simulink library "SUB_ECU_L4_MABX_HW_Interface_PTC_166"  (R2018a)
settings: Solver=VariableStepAuto  StartTime=0.0  StopTime=10.0  RelTol=1e-3
PostLoadFcn:
  | , if any(exist('dsrtsu_mdlpostloadfcn', 'file') == [2, 3, 6]), try dsrtsu_mdlpostloadfcn('Execute', bdroot); catch fprintf('Error in PostLoadFcn (dsrtsu_mdlpostloadfcn) for model "%s":\n %s\n', bdroot, lasterr); end, end,
undefined symbols (not defined in the file or in its folder): CANR_PROPB_REAX_3_13_CHANNEL_APV, CANR_PROPB_REAX_4_13_CHANNEL_APV, CANR_PROPB_XPR_1_50_CHANNEL_APV, ENUM_CAN_RX_T, ENUM_CAN_TX_T, ENUM_REAX_OPERATION_MODE_T, ENUM_SIGNAL_HEALTH_T, ENUM_XBR_CONTROL_MODE_T, ENUM_XBR_EBI_MODE_T, ENUM_XBR_PASS_THROUGH_ACTIVE_T, ENUM_XBR_PRIORITY_T, ENUM_XPR_INHIBIT_PARK_MANUAL_T, ENUM_XPR_INHIBIT_UNPARK_MANUAL_T, ENUM_XPR_PARK_MANUAL_T, ENUM_XPR_UNPARK_MANUAL_T, PROPB_REAX_1_E4_DES_POS_SIG_SRC_APV, PROPB_REAX_1_E4_DESIRED_OPMODE_APV, PROPB_REAX_1_E4_DESIRED_POSITION_APV, ptc_matlab_lib
libraries: PTC_MBDS_LIB x163, rtican x79, simulink x41, EmE_MBD_Blockset x35, rti1401lib_dio_type4 x8, simulink_need_slupdate x7, $bdroot x5, rti1401lib_adc_type4 x3, rtitasklib x1
(part 18 of 25)

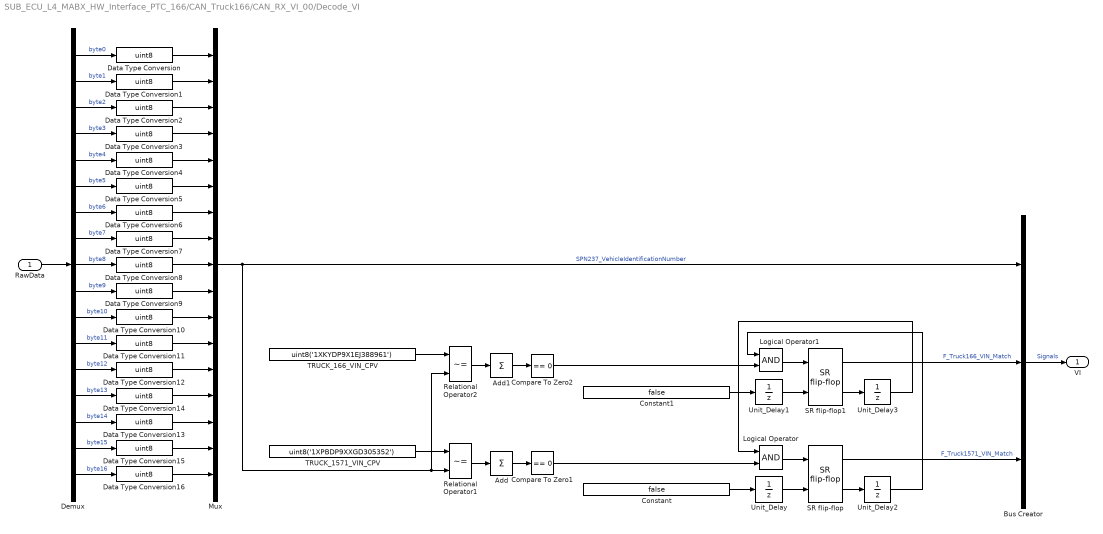
== system SUB_ECU_L4_MABX_HW_Interface_PTC_166/CAN_Truck166/CAN_RX_VI_00/Decode_VI ==
  RawData : Inport  OutDataTypeStr=uint8  PortDimensions=17
  Add : Sum  Inputs=+  InputSameDT=on
  Add1 : Sum  Inputs=+  InputSameDT=on
  Bus Creator : BusCreator  Inputs=3
  Compare To Zero1 : simulink/Logic and Bit Operations/Compare To Zero  relop===  OutDataTypeStr=boolean
  Compare To Zero2 : simulink/Logic and Bit Operations/Compare To Zero  relop===  OutDataTypeStr=boolean
  Constant : Constant  Value=false
  Constant1 : Constant  Value=false
  Data Type Conversion{,1..16} (17 alike) : DataTypeConversion  OutDataTypeStr=uint8
  Demux : Demux  Outputs=17
  Logical Operator : Logic  OutDataTypeStr=boolean
  Logical Operator1 : Logic  OutDataTypeStr=boolean
  Mux : Mux  Inputs=17
  Relational Operator1 : RelationalOperator  Operator=~=  OutDataTypeStr=boolean  RndMeth=Nearest  InputSameDT=on
  Relational Operator2 : RelationalOperator  Operator=~=  OutDataTypeStr=boolean  RndMeth=Nearest  InputSameDT=on
  SR flip-flop : EmE_MBD_Blockset/Logic and Bit Operations/SR flip-flop
      settings: SourceProductName=PACCAR EmE MBD Blockset
  SR flip-flop1 : EmE_MBD_Blockset/Logic and Bit Operations/SR flip-flop
      settings: SourceProductName=PACCAR EmE MBD Blockset
  TRUCK_1571_VIN_CPV : Constant  Value=uint8('1XPBDP9XXGD305352')
  TRUCK_166_VIN_CPV : Constant  Value=uint8('1XKYDP9X1EJ388961')
  Unit_Delay{,1..3} (4 alike) : UnitDelay  InitialCondition=true  SampleTime=-1
      settings: AttributesFormatString=IC: %<vinit>
  VI : Outport
  wires:
  Unit_Delay3/1 -> Logical Operator/1
  Unit_Delay2/1 -> Logical Operator1/1
  SR flip-flop/2 -> Unit_Delay2/1
  Compare To Zero2/1 -> Logical Operator1/2
  Logical Operator1/1 -> SR flip-flop1/1
  Logical Operator/1 -> SR flip-flop/1
  SR flip-flop1/2 -> Unit_Delay3/1
  Constant1/1 -> Unit_Delay1/1
  Unit_Delay1/1 -> SR flip-flop1/2
  Compare To Zero1/1 -> Logical Operator/2
  Constant/1 -> Unit_Delay/1
  Unit_Delay/1 -> SR flip-flop/2
  Bus Creator/1 -> VI/1  "Signals"
  Demux/17 -> Data Type Conversion16/1  "byte16"
  Demux/16 -> Data Type Conversion15/1  "byte15"
  Demux/1 -> Data Type Conversion/1  "byte0"
  Demux/15 -> Data Type Conversion13/1  "byte14"
  Demux/14 -> Data Type Conversion14/1  "byte13"
  Demux/2 -> Data Type Conversion1/1  "byte1"
  Demux/3 -> Data Type Conversion2/1  "byte2"
  Demux/13 -> Data Type Conversion12/1  "byte12"
  Demux/4 -> Data Type Conversion3/1  "byte3"
  Demux/12 -> Data Type Conversion11/1  "byte11"
  Demux/5 -> Data Type Conversion4/1  "byte4"
  Demux/11 -> Data Type Conversion10/1  "byte10"
  Demux/10 -> Data Type Conversion9/1  "byte9"
  Demux/6 -> Data Type Conversion5/1  "byte5"
  Demux/7 -> Data Type Conversion6/1  "byte6"
  Demux/9 -> Data Type Conversion8/1  "byte8"
  Demux/8 -> Data Type Conversion7/1  "byte7"
  SR flip-flop1/1 -> Bus Creator/2  "F_Truck166_VIN_Match"
  SR flip-flop/1 -> Bus Creator/3  "F_Truck1571_VIN_Match"
  Add1/1 -> Compare To Zero2/1
  Relational Operator2/1 -> Add1/1
  TRUCK_1571_VIN_CPV/1 -> Relational Operator1/1
  TRUCK_166_VIN_CPV/1 -> Relational Operator2/1
  Add/1 -> Compare To Zero1/1
  Relational Operator1/1 -> Add/1
  Data Type Conversion14/1 -> Mux/14
  Data Type Conversion4/1 -> Mux/5
  Data Type Conversion9/1 -> Mux/10
  Data Type Conversion3/1 -> Mux/4
  Data Type Conversion2/1 -> Mux/3
  Data Type Conversion15/1 -> Mux/16
  Data Type Conversion8/1 -> Mux/9
  Data Type Conversion13/1 -> Mux/15
  Data Type Conversion12/1 -> Mux/13
  Data Type Conversion7/1 -> Mux/8
  Data Type Conversion11/1 -> Mux/12
  Data Type Conversion10/1 -> Mux/11
  Data Type Conversion6/1 -> Mux/7
  Data Type Conversion1/1 -> Mux/2
  Data Type Conversion/1 -> Mux/1
  Data Type Conversion5/1 -> Mux/6
  Data Type Conversion16/1 -> Mux/17
  Mux/1 -> Bus Creator/1, Relational Operator1/2, Relational Operator2/2  "SPN237_VehicleIdentificationNumber"
  RawData/1 -> Demux/1

== system SUB_ECU_L4_MABX_HW_Interface_PTC_166/CAN_Truck166/Decode_PropB_REAX_3/decode_byte1 ==
  byte1 : Inport
  AND1 : PTC_MBDS_LIB/MBDS Standard Library/Basic Operations/Logic and Bit Operations/AND  BitwiseMode=on  Inputs=1  UseBitMask=on  BitMask=bin2dec('11110000')  OutDataTypeStr=uint8  PTC_MBDS_BlockVersion=5.41  PTC_BlockType=PTC_MBDS_AND
      settings: AttributesFormatString=bitwise  SourceProductName=PACCAR Technical Center MBDS Library
  AND2 : PTC_MBDS_LIB/MBDS Standard Library/Basic Operations/Logic and Bit Operations/AND  BitwiseMode=on  Inputs=1  UseBitMask=on  BitMask=bin2dec('00001111')  OutDataTypeStr=uint8  PTC_MBDS_BlockVersion=5.41  PTC_BlockType=PTC_MBDS_AND
      settings: AttributesFormatString=bitwise  SourceProductName=PACCAR Technical Center MBDS Library
  Bus Creator : BusCreator  Inputs=2
  "Shift_Arithmetic " : ArithShift  BitShiftNumber=4
  Out : Outport
  wires:
  Bus Creator/1 -> Out/1
  AND1/1 -> "Shift_Arithmetic "/1
  AND2/1 -> Bus Creator/1  "PropB_REAX_3_CurrentOperatingMode"
  byte1/1 -> AND2/1, AND1/1
  "Shift_Arithmetic "/1 -> Bus Creator/2  "PropB_REAX_3_ReqOperatingMode"

== system SUB_ECU_L4_MABX_HW_Interface_PTC_166/CAN_Truck166/Decode_PropB_REAX_3/decode_byte2 ==
  byte2 : Inport
  Bus Creator : BusCreator  Inputs=1
  Out : Outport
  wires:
  Bus Creator/1 -> Out/1
  byte2/1 -> Bus Creator/1  "PropB_REAX_3_StatusErrMsg"

== system SUB_ECU_L4_MABX_HW_Interface_PTC_166/CAN_Truck166/Decode_PropB_REAX_3/decode_byte3_byte4 ==
  byte3 : Inport
  byte4 : Inport  Port=2
  Bus Creator : BusCreator  Inputs=1
  Constant : Constant  Value=1/1024
  Data Type Conversion1 : DataTypeConversion  OutDataTypeStr=uint16  SaturateOnIntegerOverflow=on
  Data Type Conversion2 : DataTypeConversion  OutDataTypeStr=uint16  SaturateOnIntegerOverflow=on
  Data Type Conversion3 : DataTypeConversion  OutDataTypeStr=int16  ConvertRealWorld=Stored Integer (SI)
  Data Type Conversion4 : DataTypeConversion  SaturateOnIntegerOverflow=on
  OR : PTC_MBDS_LIB/MBDS Standard Library/Basic Operations/Logic and Bit Operations/OR  BitwiseMode=on  Inputs=2  UseBitMask=off  BitMask='A7'  OutDataTypeStr=uint16  PTC_MBDS_BlockVersion=5.41  PTC_BlockType=PTC_MBDS_OR
      settings: AttributesFormatString=bitwise  SourceProductName=PACCAR Technical Center MBDS Library
  Product : Product  Inputs=**  OutDataTypeStr=single  SaturateOnIntegerOverflow=on  InputSameDT=on
      settings: AttributesFormatString=Saturate: %<SaturateOnIntegerOverflow>
  Shift_Arithmetic 1 : ArithShift  BitShiftNumber=-8
  Out : Outport
  wires:
  Bus Creator/1 -> Out/1
  Data Type Conversion4/1 -> Product/1
  OR/1 -> Data Type Conversion3/1
  Shift_Arithmetic 1/1 -> OR/2
  Data Type Conversion1/1 -> OR/1
  Data Type Conversion2/1 -> Shift_Arithmetic 1/1
  byte4/1 -> Data Type Conversion2/1
  byte3/1 -> Data Type Conversion1/1
  Data Type Conversion3/1 -> Data Type Conversion4/1
  Constant/1 -> Product/2
  Product/1 -> Bus Creator/1  "PropB_REAX_3_HandwheelTorque"

== system SUB_ECU_L4_MABX_HW_Interface_PTC_166/CAN_Truck166/Decode_PropB_REAX_3/decode_byte5_byte6 ==
  byte5 : Inport
  byte6 : Inport  Port=2
  Bus Creator : BusCreator  Inputs=1
  Constant1 : Constant  Value=1/1024
  Data Type Conversion1 : DataTypeConversion  SaturateOnIntegerOverflow=on
  Data Type Conversion4 : DataTypeConversion  OutDataTypeStr=uint16  SaturateOnIntegerOverflow=on
  Data Type Conversion5 : DataTypeConversion  OutDataTypeStr=uint16  SaturateOnIntegerOverflow=on
  Data Type Conversion6 : DataTypeConversion  OutDataTypeStr=int16  ConvertRealWorld=Stored Integer (SI)
  OR1 : PTC_MBDS_LIB/MBDS Standard Library/Basic Operations/Logic and Bit Operations/OR  BitwiseMode=on  Inputs=2  UseBitMask=off  BitMask='A7'  OutDataTypeStr=uint16  PTC_MBDS_BlockVersion=5.41  PTC_BlockType=PTC_MBDS_OR
      settings: AttributesFormatString=bitwise  SourceProductName=PACCAR Technical Center MBDS Library
  Product1 : Product  Inputs=**  OutDataTypeStr=single  SaturateOnIntegerOverflow=on  InputSameDT=on
      settings: AttributesFormatString=Saturate: %<SaturateOnIntegerOverflow>
  Shift_Arithmetic 2 : ArithShift  BitShiftNumber=-8
  Out : Outport
  wires:
  Bus Creator/1 -> Out/1
  Data Type Conversion1/1 -> Product1/1
  Product1/1 -> Bus Creator/1  "PropB_REAX_3_HandwheelVelocity"
  Constant1/1 -> Product1/2
  Data Type Conversion6/1 -> Data Type Conversion1/1
  OR1/1 -> Data Type Conversion6/1
  Data Type Conversion4/1 -> OR1/1
  Data Type Conversion5/1 -> Shift_Arithmetic 2/1
  Shift_Arithmetic 2/1 -> OR1/2
  byte6/1 -> Data Type Conversion5/1
  byte5/1 -> Data Type Conversion4/1

== system SUB_ECU_L4_MABX_HW_Interface_PTC_166/CAN_Truck166/Decode_PropB_REAX_3/decode_byte7_byte8 ==
  byte7 : Inport
  byte8 : Inport  Port=2
  Bus Creator : BusCreator  Inputs=1
  Constant2 : Constant  Value=360/8192
  Data Type Conversion1 : DataTypeConversion  SaturateOnIntegerOverflow=on
  Data Type Conversion7 : DataTypeConversion  OutDataTypeStr=uint16  SaturateOnIntegerOverflow=on
  Data Type Conversion8 : DataTypeConversion  OutDataTypeStr=uint16  SaturateOnIntegerOverflow=on
  Data Type Conversion9 : DataTypeConversion  OutDataTypeStr=int16  ConvertRealWorld=Stored Integer (SI)
  OR2 : PTC_MBDS_LIB/MBDS Standard Library/Basic Operations/Logic and Bit Operations/OR  BitwiseMode=on  Inputs=2  UseBitMask=off  BitMask='A7'  OutDataTypeStr=uint16  PTC_MBDS_BlockVersion=5.41  PTC_BlockType=PTC_MBDS_OR
      settings: AttributesFormatString=bitwise  SourceProductName=PACCAR Technical Center MBDS Library
  Product2 : Product  Inputs=**  OutDataTypeStr=single  SaturateOnIntegerOverflow=on  InputSameDT=on
      settings: AttributesFormatString=Saturate: %<SaturateOnIntegerOverflow>
  Shift_Arithmetic 3 : ArithShift  BitShiftNumber=-8
  Out : Outport
  wires:
  Bus Creator/1 -> Out/1
  Data Type Conversion1/1 -> Product2/1
  Data Type Conversion9/1 -> Data Type Conversion1/1
  Constant2/1 -> Product2/2
  OR2/1 -> Data Type Conversion9/1
  Shift_Arithmetic 3/1 -> OR2/2
  Data Type Conversion7/1 -> OR2/1
  Data Type Conversion8/1 -> Shift_Arithmetic 3/1
  byte7/1 -> Data Type Conversion7/1
  Product2/1 -> Bus Creator/1  "PropB_REAX_3_PullCompensation"
  byte8/1 -> Data Type Conversion8/1

== system SUB_ECU_L4_MABX_HW_Interface_PTC_166/CAN_Truck166/Decode_PropB_REAX_4/decode_byte1 ==
  byte1 : Inport
  AND : PTC_MBDS_LIB/MBDS Standard Library/Basic Operations/Logic and Bit Operations/AND  BitwiseMode=on  Inputs=1  UseBitMask=on  BitMask=bin2dec('00000001')  OutDataTypeStr=boolean  PTC_MBDS_BlockVersion=5.41  PTC_BlockType=PTC_MBDS_AND
      settings: AttributesFormatString=bitwise  SourceProductName=PACCAR Technical Center MBDS Library
  AND1 : PTC_MBDS_LIB/MBDS Standard Library/Basic Operations/Logic and Bit Operations/AND  BitwiseMode=on  Inputs=1  UseBitMask=on  BitMask=bin2dec('00000010')  OutDataTypeStr=uint8  PTC_MBDS_BlockVersion=5.41  PTC_BlockType=PTC_MBDS_AND
      settings: AttributesFormatString=bitwise  SourceProductName=PACCAR Technical Center MBDS Library
  AND2 : PTC_MBDS_LIB/MBDS Standard Library/Basic Operations/Logic and Bit Operations/AND  BitwiseMode=on  Inputs=1  UseBitMask=on  BitMask=bin2dec('00000100')  OutDataTypeStr=uint8  PTC_MBDS_BlockVersion=5.41  PTC_BlockType=PTC_MBDS_AND
      settings: AttributesFormatString=bitwise  SourceProductName=PACCAR Technical Center MBDS Library
  Bus Creator : BusCreator  Inputs=3
  Data Type Conversion : DataTypeConversion  OutDataTypeStr=boolean  SaturateOnIntegerOverflow=on
  Data Type Conversion1 : DataTypeConversion  OutDataTypeStr=boolean  SaturateOnIntegerOverflow=on
  "Shift_Arithmetic " : ArithShift  BitShiftNumber=1
  Shift_Arithmetic 1 : ArithShift  BitShiftNumber=2
  Out : Outport
  wires:
  Data Type Conversion1/1 -> Bus Creator/3  "PropB_REAX_4_DriverControlledEffortsEnabled"
  Data Type Conversion/1 -> Bus Creator/2  "PropB_REAX_4_PositionIndexValid"
  Bus Creator/1 -> Out/1
  Shift_Arithmetic 1/1 -> Data Type Conversion1/1
  "Shift_Arithmetic "/1 -> Data Type Conversion/1
  AND1/1 -> "Shift_Arithmetic "/1
  byte1/1 -> AND/1, AND1/1, AND2/1
  AND2/1 -> Shift_Arithmetic 1/1
  AND/1 -> Bus Creator/1  "PropB_REAX_4_AbsSteeringPosValid"

== system SUB_ECU_L4_MABX_HW_Interface_PTC_166/CAN_Truck166/Decode_PropB_REAX_4/decode_byte2 ==
  byte2 : Inport
  Bus Creator : BusCreator  Inputs=1
  SignalConversion : SignalConversion  ConversionOutput=Contiguous copy  OverrideOpt=off
  Out : Outport
  wires:
  Bus Creator/1 -> Out/1
  SignalConversion/1 -> Bus Creator/1  "PropB_REAX_4_ControlOperatingMode"
  byte2/1 -> SignalConversion/1

== system SUB_ECU_L4_MABX_HW_Interface_PTC_166/CAN_Truck166/Decode_PropB_REAX_4/decode_byte3 ==
  byte3 : Inport
  Bus Creator : BusCreator  Inputs=1
  SignalConversion : SignalConversion  ConversionOutput=Contiguous copy  OverrideOpt=off
  Out : Outport
  wires:
  Bus Creator/1 -> Out/1
  SignalConversion/1 -> Bus Creator/1  "PropB_REAX_4_SystemMode"
  byte3/1 -> SignalConversion/1

== system SUB_ECU_L4_MABX_HW_Interface_PTC_166/CAN_Truck166/Decode_PropB_REAX_4/decode_byte5 ==
  byte5 : Inport
  Bus Creator : BusCreator  Inputs=1
  Data Type Conversion4 : DataTypeConversion  OutDataTypeStr=int8  ConvertRealWorld=Stored Integer (SI)
  Data Type Conversion5 : DataTypeConversion  OutDataTypeStr=double  SaturateOnIntegerOverflow=on
  Out : Outport
  wires:
  Bus Creator/1 -> Out/1
  Data Type Conversion5/1 -> Bus Creator/1  "PropB_REAX_4_PercHandwheelTorque"
  Data Type Conversion4/1 -> Data Type Conversion5/1
  byte5/1 -> Data Type Conversion4/1

== system SUB_ECU_L4_MABX_HW_Interface_PTC_166/CAN_Truck166/Decode_PropB_REAX_4/decode_byte6_byte7 ==
  byte6 : Inport
  byte7 : Inport  Port=2
  Bus Creator : BusCreator  Inputs=1
  Data Type Conversion6 : DataTypeConversion  OutDataTypeStr=uint16  SaturateOnIntegerOverflow=on
  Data Type Conversion7 : DataTypeConversion  OutDataTypeStr=uint16  SaturateOnIntegerOverflow=on
  Data Type Conversion8 : DataTypeConversion  OutDataTypeStr=int16  ConvertRealWorld=Stored Integer (SI)
  Data Type Conversion9 : DataTypeConversion  OutDataTypeStr=double  SaturateOnIntegerOverflow=on
  OR : PTC_MBDS_LIB/MBDS Standard Library/Basic Operations/Logic and Bit Operations/OR  BitwiseMode=on  Inputs=2  UseBitMask=off  BitMask='A7'  OutDataTypeStr=uint16  PTC_MBDS_BlockVersion=5.41  PTC_BlockType=PTC_MBDS_OR
      settings: AttributesFormatString=bitwise  SourceProductName=PACCAR Technical Center MBDS Library
  Shift_Arithmetic 2 : ArithShift  BitShiftNumber=-8
  Out : Outport
  wires:
  Bus Creator/1 -> Out/1
  OR/1 -> Data Type Conversion8/1
  Data Type Conversion8/1 -> Data Type Conversion9/1
  Shift_Arithmetic 2/1 -> OR/2
  Data Type Conversion7/1 -> Shift_Arithmetic 2/1
  Data Type Conversion6/1 -> OR/1
  byte7/1 -> Data Type Conversion7/1
  byte6/1 -> Data Type Conversion6/1
  Data Type Conversion9/1 -> Bus Creator/1  "PropB_REAX_4_AbsSteeringAngle"

== system SUB_ECU_L4_MABX_HW_Interface_PTC_166/CAN_Truck166/Decode_PropB_REAX_4/decode_byte8 ==
  byte8 : Inport
  Bus Creator : BusCreator  Inputs=1
  Data Type Conversion10 : DataTypeConversion  OutDataTypeStr=int8  ConvertRealWorld=Stored Integer (SI)
  Data Type Conversion11 : DataTypeConversion  OutDataTypeStr=double  SaturateOnIntegerOverflow=on
  Out : Outport
  wires:
  Bus Creator/1 -> Out/1
  byte8/1 -> Data Type Conversion10/1
  Data Type Conversion10/1 -> Data Type Conversion11/1
  Data Type Conversion11/1 -> Bus Creator/1  "PropB_REAX_4_PercMotorTorque"

== system SUB_ECU_L4_MABX_HW_Interface_PTC_166/DIGITAL/PWM pedal input management/Arbitrate pedal position output ==
  F_Pedal_pwm_sens_total_failure : Inport
  Pedal_synch_data_F_Hard : Inport  Port=2
  Pedal_pwm_angle_common : Inport  Port=3
  CPV : EmE_MBD_Blockset/Sources/CPV  conval=0.1
      settings: SourceProductName=PACCAR EmE MBD Blockset
  F_PEDAL_TORQUE_SLEW_AT_FAULT : Constant  Value=true
  If_Then_Else : EmE_MBD_Blockset/Signal Routing/If_Then_Else
      settings: SourceProductName=PACCAR EmE MBD Blockset
  Logical Operator1 : Logic  Operator=OR  OutDataTypeStr=boolean
  Logical Operator6 : Logic  Operator=OR  OutDataTypeStr=boolean
  PEDAL_PWM_SENSOR_DATA_APV.DEFAULT_SLEW_DOWN : Constant  Value=25
  PEDAL_PWM_SENSOR_DATA_APV.DEFAULT_SLEW_UP : Constant  Value=25
  PEDAL_PWM_SENSOR_DATA_APV.DEFAULT_VALUE : Constant  Value=0
  PEDAL_PWM_SENSOR_DATA_APV.DT : Constant  Value=0.01
  Relational Operator : EmE_MBD_Blockset/Logic and Bit Operations/Relational Operator  func=<=
      settings: SourceProductName=PACCAR EmE MBD Blockset
  SR flip-flop1 : EmE_MBD_Blockset/Logic and Bit Operations/SR flip-flop
      settings: SourceProductName=PACCAR EmE MBD Blockset
  Slew_at_event : EmE_MBD_Blockset/Math Operators/Slew_at_event
      settings: SourceProductName=PACCAR EmE MBD Blockset
  Terminator : Terminator
  Pedal_pwm_position : Outport
  DEFAULT_VALUE : Outport  Port=2
  wires:
  F_Pedal_pwm_sens_total_failure/1 -> Logical Operator6/1
  Slew_at_event/1 -> Logical Operator1/2
  CPV/1 -> Relational Operator/2
  SR flip-flop1/1 -> If_Then_Else/1
  SR flip-flop1/2 -> Terminator/1
  Logical Operator1/1 -> SR flip-flop1/1  "F_Pedal_pwm_fault_slew_enabled"
  F_PEDAL_TORQUE_SLEW_AT_FAULT/1 -> Slew_at_event/Enable
  PEDAL_PWM_SENSOR_DATA_APV.DT/1 -> Slew_at_event/6
  PEDAL_PWM_SENSOR_DATA_APV.DEFAULT_SLEW_DOWN/1 -> Slew_at_event/5
  Relational Operator/1 -> SR flip-flop1/2
  Logical Operator6/1 -> Logical Operator1/1, Slew_at_event/1
  Slew_at_event/2 -> If_Then_Else/2  "Pedal_pwm_angle_common_slewed"
  If_Then_Else/1 -> Pedal_pwm_position/1  "Pedal_pwm_position"
  Pedal_pwm_angle_common/1 -> If_Then_Else/3, Relational Operator/1, Slew_at_event/2
  Pedal_synch_data_F_Hard/1 -> Logical Operator6/2
  PEDAL_PWM_SENSOR_DATA_APV.DEFAULT_SLEW_UP/1 -> Slew_at_event/4
  PEDAL_PWM_SENSOR_DATA_APV.DEFAULT_VALUE/1 -> Slew_at_event/3, DEFAULT_VALUE/1

== system SUB_ECU_L4_MABX_HW_Interface_PTC_166/DIGITAL/PWM pedal input management/Determine common angle ==
  Pedal_1_pwm_health_state : Inport
  F_Pedal_pwm_sens_total_failure : Inport  Port=2
  Pedal_2_pwm_health_state : Inport  Port=3
  Pedal_1_pwm_angle_arbitrated : Inport  Port=4
  Pedal_2_pwm_angle_arbitrated : Inport  Port=5
  DEFAULT_VALUE : Inport  Port=6
  Compare To Constant1 : simulink/Logic and Bit Operations/Compare To Constant  relop===  const=ENUM_SIGNAL_HEALTH_T.FAULT_ACTIVE  OutDataTypeStr=boolean
  Compare To Constant3 : simulink/Logic and Bit Operations/Compare To Constant  relop===  const=ENUM_SIGNAL_HEALTH_T.FAULT_ACTIVE  OutDataTypeStr=boolean
  If_Then_Else : EmE_MBD_Blockset/Signal Routing/If_Then_Else
      settings: SourceProductName=PACCAR EmE MBD Blockset
  If_Then_Else1 : EmE_MBD_Blockset/Signal Routing/If_Then_Else
      settings: SourceProductName=PACCAR EmE MBD Blockset
  If_Then_Else2 : EmE_MBD_Blockset/Signal Routing/If_Then_Else
      settings: SourceProductName=PACCAR EmE MBD Blockset
  MinMax : MinMax  Inputs=2  InputSameDT=on
  Pedal_pwm_angle_common : Outport
  wires:
  F_Pedal_pwm_sens_total_failure/1 -> If_Then_Else/1
  Pedal_2_pwm_angle_arbitrated/1 -> If_Then_Else2/3, If_Then_Else1/2
  DEFAULT_VALUE/1 -> If_Then_Else/2
  If_Then_Else/1 -> Pedal_pwm_angle_common/1  "Pedal_pwm_angle_common"
  Pedal_1_pwm_health_state/1 -> Compare To Constant3/1
  Pedal_2_pwm_health_state/1 -> Compare To Constant1/1
  Compare To Constant3/1 -> If_Then_Else1/1
  Pedal_1_pwm_angle_arbitrated/1 -> If_Then_Else2/2, If_Then_Else1/3
  Compare To Constant1/1 -> If_Then_Else2/1
  If_Then_Else2/1 -> MinMax/2  "Pedal_2_pwm_corr"
  If_Then_Else1/1 -> MinMax/1  "Pedal_1_pwm_corr"
  MinMax/1 -> If_Then_Else/3

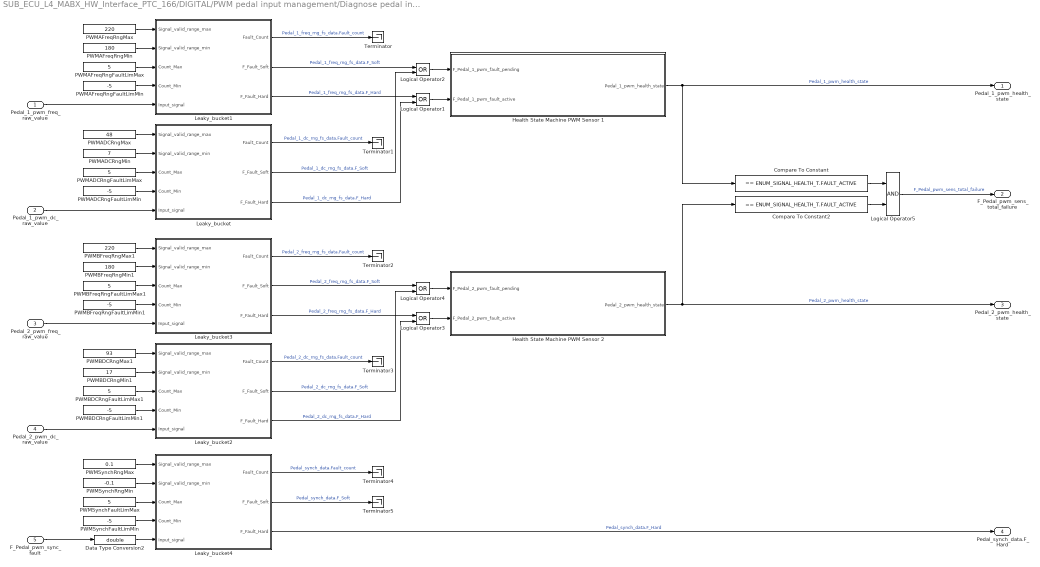
== system SUB_ECU_L4_MABX_HW_Interface_PTC_166/DIGITAL/PWM pedal input management/Diagnose pedal input signals ==
  Pedal_1_pwm_freq_raw_value : Inport
  Pedal_1_pwm_dc_raw_value : Inport  Port=2
  Pedal_2_pwm_freq_raw_value : Inport  Port=3
  Pedal_2_pwm_dc_raw_value : Inport  Port=4
  F_Pedal_pwm_sync_fault : Inport  Port=5
  Compare To Constant : simulink/Logic and Bit Operations/Compare To Constant  relop===  const=ENUM_SIGNAL_HEALTH_T.FAULT_ACTIVE  OutDataTypeStr=boolean
  Compare To Constant2 : simulink/Logic and Bit Operations/Compare To Constant  relop===  const=ENUM_SIGNAL_HEALTH_T.FAULT_ACTIVE  OutDataTypeStr=boolean
  Data Type Conversion2 : DataTypeConversion  OutDataTypeStr=double  SaturateOnIntegerOverflow=on
  Health State Machine PWM Sensor 1 : Stateflow chart  TreatAsAtomicUnit=on
  Health State Machine PWM Sensor 2 : Stateflow chart  TreatAsAtomicUnit=on
  Leaky_bucket : Subsystem
  Leaky_bucket1 : Subsystem
  Leaky_bucket2 : Subsystem
  Leaky_bucket3 : Subsystem
  Leaky_bucket4 : Subsystem
  Logical Operator{1..4} (4 alike) : Logic  Operator=OR  OutDataTypeStr=boolean
  Logical Operator5 : Logic  OutDataTypeStr=boolean
  PWMADCRngFaultLimMax : Constant  Value=5
  PWMADCRngFaultLimMin : Constant  Value=-5
  PWMADCRngMax : Constant  Value=48
  PWMADCRngMin : Constant  Value=7
  PWMAFreqRngFaultLimMax : Constant  Value=5
  PWMAFreqRngFaultLimMin : Constant  Value=-5
  PWMAFreqRngMax : Constant  Value=220
  PWMAFreqRngMin : Constant  Value=180
  PWMBDCRngFaultLimMax1 : Constant  Value=5
  PWMBDCRngFaultLimMin1 : Constant  Value=-5
  PWMBDCRngMax1 : Constant  Value=93
  PWMBDCRngMin1 : Constant  Value=17
  PWMBFreqRngFaultLimMax1 : Constant  Value=5
  PWMBFreqRngFaultLimMin1 : Constant  Value=-5
  PWMBFreqRngMax1 : Constant  Value=220
  PWMBFreqRngMin1 : Constant  Value=180
  PWMSynchFaultLimMax : Constant  Value=5
  PWMSynchFaultLimMin : Constant  Value=-5
  PWMSynchRngMax : Constant  Value=0.1
  PWMSynchRngMin : Constant  Value=-0.1
  Terminator{,1..5} (6 alike) : Terminator
  Pedal_1_pwm_health_state : Outport
  F_Pedal_pwm_sens_total_failure : Outport  Port=2
  Pedal_2_pwm_health_state : Outport  Port=3
  Pedal_synch_data.F_Hard : Outport  Port=4
  wires:
  Pedal_1_pwm_freq_raw_value/1 -> Leaky_bucket1/5(Input_signal)
  Data Type Conversion2/1 -> Leaky_bucket4/5(Input_signal)
  Leaky_bucket1/3(F_Fault_Hard) -> Logical Operator1/1  "Pedal_1_freq_rng_fs_data.F_Hard"
  Leaky_bucket1/2(F_Fault_Soft) -> Logical Operator2/1  "Pedal_1_freq_rng_fs_data.F_Soft"
  PWMADCRngMax/1 -> Leaky_bucket/1(Signal_valid_range_max)
  PWMADCRngMin/1 -> Leaky_bucket/2(Signal_valid_range_min)
  PWMADCRngFaultLimMax/1 -> Leaky_bucket/3(Count_Max)
  PWMADCRngFaultLimMin/1 -> Leaky_bucket/4(Count_Min)
  Leaky_bucket/3(F_Fault_Hard) -> Logical Operator1/2  "Pedal_1_dc_rng_fs_data.F_Hard"
  Leaky_bucket/1(Fault_Count) -> Terminator1/1  "Pedal_1_dc_rng_fs_data.Fault_count"
  Leaky_bucket/2(F_Fault_Soft) -> Logical Operator2/2  "Pedal_1_dc_rng_fs_data.F_Soft"
  PWMAFreqRngMin/1 -> Leaky_bucket1/2(Signal_valid_range_min)
  PWMAFreqRngMax/1 -> Leaky_bucket1/1(Signal_valid_range_max)
  PWMAFreqRngFaultLimMax/1 -> Leaky_bucket1/3(Count_Max)
  PWMAFreqRngFaultLimMin/1 -> Leaky_bucket1/4(Count_Min)
  Leaky_bucket1/1(Fault_Count) -> Terminator/1  "Pedal_1_freq_rng_fs_data.Fault_count"
  Logical Operator1/1 -> Health State Machine PWM Sensor 1/2(F_Pedal_1_pwm_fault_active)
  Logical Operator2/1 -> Health State Machine PWM Sensor 1/1(F_Pedal_1_pwm_fault_pending)
  Leaky_bucket3/3(F_Fault_Hard) -> Logical Operator3/1  "Pedal_2_freq_rng_fs_data.F_Hard"
  Leaky_bucket3/2(F_Fault_Soft) -> Logical Operator4/1  "Pedal_2_freq_rng_fs_data.F_Soft"
  Health State Machine PWM Sensor 2/1(Pedal_2_pwm_health_state) -> Pedal_2_pwm_health_state/1, Compare To Constant2/1  "Pedal_2_pwm_health_state"
  PWMBDCRngMax1/1 -> Leaky_bucket2/1(Signal_valid_range_max)
  PWMBDCRngMin1/1 -> Leaky_bucket2/2(Signal_valid_range_min)
  PWMBDCRngFaultLimMax1/1 -> Leaky_bucket2/3(Count_Max)
  PWMBDCRngFaultLimMin1/1 -> Leaky_bucket2/4(Count_Min)
  Leaky_bucket2/3(F_Fault_Hard) -> Logical Operator3/2  "Pedal_2_dc_rng_fs_data.F_Hard"
  Leaky_bucket2/1(Fault_Count) -> Terminator3/1  "Pedal_2_dc_rng_fs_data.Fault_count"
  Leaky_bucket2/2(F_Fault_Soft) -> Logical Operator4/2  "Pedal_2_dc_rng_fs_data.F_Soft"
  PWMBFreqRngMin1/1 -> Leaky_bucket3/2(Signal_valid_range_min)
  PWMBFreqRngMax1/1 -> Leaky_bucket3/1(Signal_valid_range_max)
  PWMBFreqRngFaultLimMax1/1 -> Leaky_bucket3/3(Count_Max)
  PWMBFreqRngFaultLimMin1/1 -> Leaky_bucket3/4(Count_Min)
  Leaky_bucket3/1(Fault_Count) -> Terminator2/1  "Pedal_2_freq_rng_fs_data.Fault_count"
  Logical Operator3/1 -> Health State Machine PWM Sensor 2/2(F_Pedal_2_pwm_fault_active)
  Logical Operator4/1 -> Health State Machine PWM Sensor 2/1(F_Pedal_2_pwm_fault_pending)
  Health State Machine PWM Sensor 1/1(Pedal_1_pwm_health_state) -> Pedal_1_pwm_health_state/1, Compare To Constant/1  "Pedal_1_pwm_health_state"
  Compare To Constant/1 -> Logical Operator5/1
  Compare To Constant2/1 -> Logical Operator5/2
  Logical Operator5/1 -> F_Pedal_pwm_sens_total_failure/1  "F_Pedal_pwm_sens_total_failure"
  PWMSynchRngMax/1 -> Leaky_bucket4/1(Signal_valid_range_max)
  PWMSynchRngMin/1 -> Leaky_bucket4/2(Signal_valid_range_min)
  PWMSynchFaultLimMax/1 -> Leaky_bucket4/3(Count_Max)
  F_Pedal_pwm_sync_fault/1 -> Data Type Conversion2/1
  PWMSynchFaultLimMin/1 -> Leaky_bucket4/4(Count_Min)
  Leaky_bucket4/3(F_Fault_Hard) -> Pedal_synch_data.F_Hard/1  "Pedal_synch_data.F_Hard"
  Leaky_bucket4/1(Fault_Count) -> Terminator4/1  "Pedal_synch_data.Fault_count"
  Leaky_bucket4/2(F_Fault_Soft) -> Terminator5/1  "Pedal_synch_data.F_Soft"
  Pedal_1_pwm_dc_raw_value/1 -> Leaky_bucket/5(Input_signal)
  Pedal_2_pwm_freq_raw_value/1 -> Leaky_bucket3/5(Input_signal)
  Pedal_2_pwm_dc_raw_value/1 -> Leaky_bucket2/5(Input_signal)

== system SUB_ECU_L4_MABX_HW_Interface_PTC_166/DIGITAL/PWM pedal input management/Fault arbitration ==
  Pedal_1_pwm_health_state : Inport
  Pedal_1_pwm_undefault : Inport  Port=2
  DEFAULT_VALUE : Inport  Port=3
  Pedal_2_pwm_health_state : Inport  Port=4
  Pedal_2_pwm_undefault : Inport  Port=5
  Compare To Constant1 : simulink/Logic and Bit Operations/Compare To Constant  relop===  const=ENUM_SIGNAL_HEALTH_T.FAULT_PENDING  OutDataTypeStr=boolean
  Compare To Constant3 : simulink/Logic and Bit Operations/Compare To Constant  relop===  const=ENUM_SIGNAL_HEALTH_T.FAULT_ACTIVE  OutDataTypeStr=boolean
  Compare To Constant4 : simulink/Logic and Bit Operations/Compare To Constant  relop===  const=ENUM_SIGNAL_HEALTH_T.FAULT_PENDING  OutDataTypeStr=boolean
  Compare To Constant5 : simulink/Logic and Bit Operations/Compare To Constant  relop===  const=ENUM_SIGNAL_HEALTH_T.FAULT_ACTIVE  OutDataTypeStr=boolean
  If_Then_Else{,1..3} (4 alike) : EmE_MBD_Blockset/Signal Routing/If_Then_Else
      settings: SourceProductName=PACCAR EmE MBD Blockset
  Logical Operator{5..8} (4 alike) : Logic  Operator=NOT  OutDataTypeStr=boolean
  Unit Delay External IC : simulink_need_slupdate/Unit Delay External IC  tsamp=-1
      settings: SourceProductName=Simulink  SourceProductBaseCode=SL
  Unit Delay External IC1 : simulink_need_slupdate/Unit Delay External IC  tsamp=-1
      settings: SourceProductName=Simulink  SourceProductBaseCode=SL
  Pedal_1_pwm_angle_arbitrated : Outport
  Pedal_2_pwm_angle_arbitrated : Outport  Port=2
  wires:
  If_Then_Else/1 -> Pedal_1_pwm_angle_arbitrated/1  "Pedal_1_pwm_angle_arbitrated"
  DEFAULT_VALUE/1 -> [DEFAULT_VALUE], Unit Delay External IC/2, If_Then_Else/3
  Pedal_1_pwm_undefault/1 -> If_Then_Else1/2
  If_Then_Else1/1 -> If_Then_Else/2, Unit Delay External IC/1
  Logical Operator7/1 -> If_Then_Else2/1
  Pedal_2_pwm_undefault/1 -> If_Then_Else3/2
  Pedal_2_pwm_health_state/1 -> Compare To Constant5/1, Compare To Constant4/1
  Logical Operator6/1 -> If_Then_Else1/1
  If_Then_Else3/1 -> Unit Delay External IC1/1, If_Then_Else2/2
  Pedal_1_pwm_health_state/1 -> Compare To Constant1/1, Compare To Constant3/1
  Compare To Constant3/1 -> Logical Operator5/1
  Logical Operator5/1 -> If_Then_Else/1
  Compare To Constant1/1 -> Logical Operator6/1
  Compare To Constant5/1 -> Logical Operator7/1
  Unit Delay External IC/1 -> If_Then_Else1/3
  Unit Delay External IC1/1 -> If_Then_Else3/3
  If_Then_Else2/1 -> Pedal_2_pwm_angle_arbitrated/1  "Pedal_2_pwm_angle_arbitrated"
  [DEFAULT_VALUE] -> If_Then_Else2/3, Unit Delay External IC1/2
  Logical Operator8/1 -> If_Then_Else3/1
  Compare To Constant4/1 -> Logical Operator8/1

== system SUB_ECU_L4_MABX_HW_Interface_PTC_166/DIGITAL/PWM pedal input management/PWM signal filtering conversion ==
  Pedal _1_pwm_dc_raw_value : Inport
  Pedal _2_pwm_dc_raw_value : Inport  Port=2
  Constant : Constant  Value=false
  Constant1 : Constant  Value=false
  LPF_first_order : EmE_MBD_Blockset/Discrete/LPF_first_order
      settings: SourceProductName=PACCAR EmE MBD Blockset
  LPF_first_order1 : EmE_MBD_Blockset/Discrete/LPF_first_order
      settings: SourceProductName=PACCAR EmE MBD Blockset
  PEDAL_PWM_ANGLE_SENS_1_MPV : Lookup_n-D  NumberOfTableDimensions=1  BreakpointsForDimension1=[0 10 20 45 90 91 99.5 100]  Table=[-25 0 28.57 100 228.57 231.43 255 255]  ExtrapMethod=Clip  UseLastTableValue=on  InputSameDT=on
      settings: AttributesFormatString=|
      | X: %<BreakpointsForDimension1>
      | Y: %<Table>
  PEDAL_PWM_ANGLE_SENS_2_MPV : Lookup_n-D  NumberOfTableDimensions=1  BreakpointsForDimension1=[0 10 20 45 90 91 99.5 100]  Table=[-25 -14.29 0 35.71 100 101.43 113.57 114.29]  ExtrapMethod=Clip  UseLastTableValue=on  InputSameDT=on
      settings: AttributesFormatString=|
      | X: %<BreakpointsForDimension1>
      | Y: %<Table>
  PEDAL_PWM_SENSOR_DATA_APV.T1_CONST : Constant  Value=0.1
  PEDAL_PWM_SENSOR_DATA_APV.T2_CONST : Constant  Value=0.1
  Unit_Delay : UnitDelay  InitialCondition=true  SampleTime=-1
      settings: AttributesFormatString=IC: %<vinit>
  Unit_Delay1 : UnitDelay  InitialCondition=true  SampleTime=-1
      settings: AttributesFormatString=IC: %<vinit>
  dT : Constant  Value=0.01
  dT1 : Constant  Value=0.01
  Pedal_1_pwm_undefault : Outport
  Pedal_2_pwm_undefault : Outport  Port=2
  wires:
  Unit_Delay/1 -> LPF_first_order/1
  PEDAL_PWM_SENSOR_DATA_APV.T1_CONST/1 -> LPF_first_order/4
  Pedal _1_pwm_dc_raw_value/1 -> LPF_first_order/2, LPF_first_order/3
  Constant/1 -> Unit_Delay/1
  dT/1 -> LPF_first_order/5
  LPF_first_order/1 -> PEDAL_PWM_ANGLE_SENS_1_MPV/1
  Unit_Delay1/1 -> LPF_first_order1/1
  PEDAL_PWM_SENSOR_DATA_APV.T2_CONST/1 -> LPF_first_order1/4
  Pedal _2_pwm_dc_raw_value/1 -> LPF_first_order1/3, LPF_first_order1/2
  Constant1/1 -> Unit_Delay1/1
  dT1/1 -> LPF_first_order1/5
  LPF_first_order1/1 -> PEDAL_PWM_ANGLE_SENS_2_MPV/1
  PEDAL_PWM_ANGLE_SENS_2_MPV/1 -> Pedal_2_pwm_undefault/1  "Pedal_2_pwm_undefault"
  PEDAL_PWM_ANGLE_SENS_1_MPV/1 -> Pedal_1_pwm_undefault/1  "Pedal_1_pwm_undefault"

== system SUB_ECU_L4_MABX_HW_Interface_PTC_166/DIGITAL/PWM pedal input management/Synchronization check sensor 1 and 2 ==
  Pedal_pwm_angle_common : Inport
  Pedal_1_pwm_undefault : Inport  Port=2
  Pedal_2_pwm_undefault : Inport  Port=3
  Abs : Abs
  PEDAL_PWM_ANGLE_DEV_MPV : Lookup_n-D  NumberOfTableDimensions=1  BreakpointsForDimension1=[0 14 15 20 80 85 86 100]  Table=[10 10 10 10 10 10 10 10]  ExtrapMethod=Clip  UseLastTableValue=on  InputSameDT=on
      settings: AttributesFormatString=|
      | X: %<BreakpointsForDimension1>
      | Y: %<Table>
  Relational Operator : RelationalOperator  Operator=>  OutDataTypeStr=boolean  RndMeth=Nearest
  Subtract : Sum  Inputs=+-  InputSameDT=on
  F_Pedal_pwm_sync_fault : Outport
  wires:
  Pedal_2_pwm_undefault/1 -> Subtract/2
  Pedal_1_pwm_undefault/1 -> Subtract/1
  Subtract/1 -> Abs/1
  Abs/1 -> Relational Operator/1
  Relational Operator/1 -> F_Pedal_pwm_sync_fault/1  "F_Pedal_pwm_sync_fault"
  Pedal_pwm_angle_common/1 -> PEDAL_PWM_ANGLE_DEV_MPV/1
  PEDAL_PWM_ANGLE_DEV_MPV/1 -> Relational Operator/2

== system SUB_ECU_L4_MABX_HW_Interface_PTC_166/INPUTS_PTC_166/Timer_Access/IncrementTimer ==
  Function : TriggerPort  TriggerType=function-call  VariantControl=(inherit)
      settings: AttributesFormatString=States when enabling: %<StatesWhenEnabling>
  Add : Sum  OutDataTypeStr=Inherit: Inherit via back propagation  SaturateOnIntegerOverflow=on  InputSameDT=on
      settings: AttributesFormatString=Saturate: %<SaturateOnIntegerOverflow>
  Constant1 : PTC_MBDS_LIB/Extras/Sources/Constant  Value2=ptc_matlab_lib.get_system_sample_time()  PTC_MBDS_BlockVersion=5.41  PTC_BlockType=PTC_MBDS_Constant
      settings: SourceProductName=PACCAR Technical Center MBDS Library
  Unit_Delay : UnitDelay  InitialCondition=-ptc_matlab_lib.get_system_sample_time()  SampleTime=-1
      settings: AttributesFormatString=Init = %<InitialCondition>
  Out1 : Outport
      settings: AttributesFormatString=Output when disabled: %<OutputWhenDisabled>
  wires:
  Constant1/1 -> Add/1
  Add/1 -> Unit_Delay/1, Out1/1
  Unit_Delay/1 -> Add/2

== system SUB_ECU_L4_MABX_HW_Interface_PTC_166/CAN_Out_PTC_166/CAN_TX_1000ms/CAN_TX_AIR1_31/TX_CAN4 ==
  Enable : Inport
  Data : Inport  Port=2
  AIR1 : rtican/RTICAN Transmit (TX)   Reserved1=[]  Reserved2=[]  Reserved3=[]  Reserved4=[]  SfcnMessage=[]  Msg_Struct=[]  BoardTypeNo=[]  BoardNo=[]  ChannelNo=[]  Parameters=[]  DialogFcn=[]  UnitName=[]  Revision=[]  UnitValues=[]  DSProperties=struct('RTI',struct('Version',uint32(5),'BlockType',struct('isSLSource',uint8(1),'isSLSink',uint8(1),'isHWSource',uint8(0),'isHWSink',uint8(0),'isSetup',uint8(0),'isInline',uint8(1),'isNonInline',uint8(0),'isInterrupt',uint8(0),'isChannelwise',uint8(0)),'IOBoardType','RTICAN','UnitType','MESSAGE','Identifier','TX','DialogType','MSVC','BlockSet','RTICAN','SlaveProcessor','CAN'))  RTIBlockInterface=struct('InputPortsWidth',int32([1 1 1 1 1 1 1 1]),'InputPortsActive',[1 1 1 1 1 1 1 1],'InputPortsName',{{'PneumaticSupplyPress','ParkingAnd_orTrailerAirPress','ServiceBrakeCircuit1AirPress','ServiceBrakeCircuit2AirPress','AuxEquipmentSupplyPress','AirSuspensionSupplyPress','AirCompressorStatus','PowertrainCircuitAirSupplyPress'}},'InputPortsDataType',{{'SS_DOUBLE','SS_DOUBLE','SS_DOUBLE','SS_DOUBLE','SS_DOUBLE','SS_DOUBLE','SS_DOUBLE','SS_DOUBLE'}},'OutputPortsWidth',int32([1 1 1 1]),'OutputPortsActive',[1 1 1 1],'OutputPortsName',{{['TX status'],['TX time'],['TX delta time'],['TX delay time']}},'DialogFcn','rtican_message_interface_gui','BlockDisplay',{{'','center'}},'IconTransparency','on','InitLevel',3,'BlockName',struct('Token',{{'AIR1'}}),'SampleTime',{{-1}},'TriggerPort',{{'none'}},'EnablePort',{{'yes'}})  RTIBlockParameters="struct('BoardTypeNo',{{1,'OFF',[]}},'BoardNo',{{2,'ON',[1 16]}},'ChannelNo',{{2,'ON',[1 2]}},'Parameters',{{struct('DataFileSupport',struct('DataFileSelectedMaster',1,'DataFileSelectedLocal',0,'DataFileName',['c:\\data\\svn\\truck1571\\dbc\\mabx_can4.dbc|c:\\data\\svn\\svn\\powertrainsys\\trunk\\src\\projects_rcp\\my2017_rcp\\dbc files\\j1939.dbc|'],'DataFileDate',{{{['10-Feb-2017 15:17:28']},{['24-Aug-2017 12:01:59']}}},'SelectedFile',['<no file selected>']),'Options',struct('StatusSelected',1,'TimeSelected',1,'DeltaTimeSelected',1,'DelayTimeSelected',1,'DelayTimeTXCommandSelected',0,'EncodeSetUnusedBitsToOne',1,'EnableMsgLoopback',0,'TriggerPort',struct('Selected',0,'TriggerType',0),'EnablePortSelected',1,'SignalOnPortnameSelected',1,'UserCoding',struct('Selected',0,'InterfaceFile','UserEncodingFile','FcnName','UserEncodeFcn','InportSelected',0,'InportWidth',1,'OutportSelected',0,'OutportWidth',1),'TerminationMsg',struct('Selected',0,'Byte0_7','0'),'InitialMsg',struct('Selected',0,'Byte0_7','0')),'Message',struct('MsgOnBlocknameSelected',1,'MsgName','AIR1','MsgIdFormat',1,'MsgId',419343921,'MsgLength',8,'NumSignals',8,'SampleTime',-1,'StartTime',struct('Selected',0,'Value',0),'AutoRepeatTime',struct('Selected',0,'Value',1),'Timeout',struct('Selected',0,'Value',0.1),'DelayTime',struct('Selected',0,'Value',0.1),'Signal',struct('SgnName',{'PneumaticSupplyPress','ParkingAnd_orTrailerAirPress','ServiceBrakeCircuit1AirPress','ServiceBrakeCircuit2AirPress','AuxEquipmentSupplyPress','AirSuspensionSupplyPress','AirCompressorStatus','PowertrainCircuitAirSupplyPress'},'SgnStartBit',{0,8,16,24,32,40,48,56},'SgnLength',{8,8,8,8,8,8,2,8},'SgnType',{0,0,0,0,0,0,0,0},'ModeValue',{-1,-1,-1,-1,-1,-1,-1,-1},'DataType',{0,0,0,0,0,0,0,0},'ByteLayout',{0,0,0,0,0,0,0,0},'Factor',{8,8,8,8,8,8,1,8},'Offset',{0,0,0,0,0,0,0,0},'SgnComment',{{['The pneumatic pressure in the main reservoir, sometimes referred to as the wet tank.']},{['The pneumatic pressure in the circuit or reservoir for the parking brake and/or the trailer supply.']},{['The pneumatic pressure in the primary service brake circuit or reservoir, supplying the rear axle.']},{['The pneumatic pressure in the secondary service brake circuit or reservoir, supplying the front axle.']},{['The pneumatic pressure in the auxiliary circuit.']},{['The pneumatic pressure in the circuit for the electronically controlled air suspension system.']},{['Indicates whether the air compressor is actively compressing air.  ' char(10) '' char(10) '00     Compressor not active' char(10) '01     Compressor active' char(10) '10     Error indicator' char(10) '11     Not available']},{['Supply pressure to carry the pressure information for the powertrain circuit. This circuit typically would feed powertrain components such as throttles, gearbox actuators and aftertreatment actuators for EGR and SCR systems.']}},'SgnUnit',{'kPa','kPa','kPa','kPa','kPa','kPa','','kPa'},'Min',{0,0,0,0,0,0,0,0},'Max',{2000,2000,2000,2000,2000,2000,3,2000},'SLDataType',{'SS_DOUBLE','SS_DOUBLE','SS_DOUBLE','SS_DOUBLE','SS_DOUBLE','SS_DOUBLE','SS_DOUBLE','SS_DOUBLE'}),'MsgIdNumFormat',1,'MsgComment',{{['Air Supply Pressure' char(10) 'Air Supply Pressure']}}),'Version',1.2,'general',struct('isFromLib',0)),'OFF',[]}},'GroupId',{{struct('Group',{{'RTICAN'}},'No',4,'Behavior',{{'NAMECHANGE'}},'BlockType',{{'SINK'}},'NameChangeFlag',0),'OFF',[]}},'SFcnRTICANMessage',{{struct('MsgType','TX','SFcnPortType','Scalar','MsgName','AIR1','MsgIdFormat','XTD','MsgId',419343921,'MsgLength',8,'NumSignals',8,'SampleTime',-1,'StartTime',struct('Selected','no','Value',0),'AutoRepeatTime',struct('Selected','no','Value',1),'Timeout',struct('Selected','no','Value',0.1),'Signal',struct('SgnName',{'PneumaticSupplyPress','ParkingAnd_orTrailerAirPress','ServiceBrakeCircuit1AirPress','ServiceBrakeCircuit2AirPress','AuxEquipmentSupplyPress','AirSuspensionSupplyPress','AirCompressorStatus','PowertrainCircuitAirSupplyPress'},'SgnStartBit',{0,8,16,24,32,40,48,56},'SgnLength',{8,8,8,8,8,8,2,8},'SgnType',{'standard','standard','standard','standard','standard','standard','standard','standard'},'ModeValue',{-1,-1,-1,-1,-1,-1,-1,-1},'DataType',{['unsigned int'],['unsigned int'],['unsigned int'],['unsigned int'],['unsigned int'],['unsigned int'],['unsigned int'],['unsigned int']},'ByteLayout',{['little endian'],['little endian'],['little endian'],['little endian'],['little endian'],['little endian'],['little endian'],['little endian']},'Factor',{8,8,8,8,8,8,1,8},'Offset',{0,0,0,0,0,0,0,0},'SLDataType',{'SS_DOUBLE','SS_DOUBLE','SS_DOUBLE','SS_DOUBLE','SS_DOUBLE','SS_DOUBLE','SS_DOUBLE','SS_DOUBLE'}),'StatusSelected','yes','TimeSelected','yes','DeltaTimeSelected','yes','DelayTimeSelected','yes','DelayTimeTXCommandSelected','no','EncodeSetUnusedBitsToOne','yes','EnableMsgLoopback','no','TriggerPort',struct('Selected','no','TriggerType',0),'EnablePortSelected','yes','UserCoding',struct('Selected','no','InterfaceFile','UserEncodingFile','FcnName','UserEncodeFcn','InportSelected','no','InportWidth',1,'OutportSelected','no','OutportWidth',1),'TerminationMsg',struct('Selected','no','Byte0','0x00','Byte1','0x00','Byte2','0x00','Byte3','0x00','Byte4','0x00','Byte5','0x00','Byte6','0x00','Byte7','0x00'),'InitialMsg',struct('Selected','no','Byte0','0x00','Byte1','0x00','Byte2','0x00','Byte3','0x00','Byte4','0x00','Byte5','0x00','Byte6','0x00','Byte7','0x00'),'BoardType','DS1','BoardNo',2,'ControllerNo',2),'OFF',[]}},'TLCFileName',{{'rtican_tx_message','OFF',[]}})"  RTISFcnParameters=struct('SFcnRTICANMessage','struct','TLCFileName','char')  RTIBlockParaDefault=struct('BoardTypeNo',4302,'BoardNo',1,'ChannelNo',1,'Parameters',struct('DataFileSupport',struct('DataFileSelectedMaster',0,'DataFileSelectedLocal',0,'DataFileName','','DataFileDate','','SelectedFile',['<no file selected>']),'Options',struct('StatusSelected',1,'TimeSelected',1,'DeltaTimeSelected',1,'DelayTimeSelected',1,'DelayTimeTXCommandSelected',0,'EncodeSetUnusedBitsToOne',0,'EnableMsgLoopback',0,'TriggerPort',struct('Selected',0,'TriggerType','rising'),'EnablePortSelected',0,'SignalOnPortnameSelected',1,'UserCoding',struct('Selected',0,'InterfaceFile','UserEncodingFile','FcnName','UserEncodeFcn','InportSelected',0,'InportWidth',1,'OutportSelected',0,'OutportWidth',1),'TerminationMsg',struct('Selected',0,'Byte0_7','0'),'InitialMsg',struct('Selected',0,'Byte0_7','0')),'Message',struct('MsgOnBlocknameSelected',0,'MsgName',['TX Message'],'MsgIdFormat',0,'MsgId',100,'MsgLength',8,'NumSignals',1,'SampleTime',-1,'StartTime',struct('Selected',0,'Value',0),'AutoRepeatTime',struct('Selected',0,'Value',0.1),'Timeout',struct('Selected',0,'Value',0.1),'DelayTime',struct('Selected',0,'Value',0.1),'Signal',struct('SgnName',['TX signal'],'SgnStartBit',0,'SgnLength',8,'SgnType',0,'ModeValue',-1,'DataType',0,'SLDataType','SS_DOUBLE','ByteLayout',0,'Factor',1,'Offset',0,'Min',0,'Max',255,'SgnComment',{{}},'SgnUnit',''),'MsgIdNumFormat',0,'MsgComment',{{''}}),'Version',1.2,'general',struct('isFromLib',1)),'GroupId',struct('Group',{{'RTICAN'}},'No',1,'Behavior',{{'NAMECHANGE'}},'BlockType',{{'SINK'}},'NameChangeFlag',0),'SFcnRTICANMessage',struct('MsgType','TX','MsgName',['TX Message'],'MsgIdFormat','STD','MsgId',100,'MsgLength',2,'NumSignals',1,'SampleTime',-1,'StartTime',struct('Selected','no','Value',0),'AutoRepeatTime',struct('Selected','no','Value',0.1),'Timeout',struct('Selected','no','Value',0.1),'DelayTime',struct('Selected','no','Value',0.1),'Signal',struct('SgnName',['TX signal'],'SgnStartBit',0,'SgnLength',8,'SgnType','standard','ModeValue',-1,'DataType',['unsigned int'],'ByteLayout',['little endian'],'SLDataType','SS_DOUBLE','Factor',1,'Offset',0),'StatusSelected','yes','TimeSelected','yes','DeltaTimeSelected','yes','DelayTimeSelected','yes','EnablePortSelected','no','EnableMsgLoopback','no','DelayTimeTXCommandSelected','no','EncodeSetUnusedBitsToOne','no','UserCoding',struct('Selected','no','InterfaceFile','UserDecodingFile','FcnName','UserDecodeFcn','InportSelected','no','InportWidth',1,'OutportSelected','no','OutportWidth',1),'TerminationMsg',struct('Selected','no','Byte0','0x00','Byte1','0x00','Byte2','0x00','Byte3','0x00','Byte4','0x00','Byte5','0x00','Byte6','0x00','Byte7','0x00'),'InitialMsg',struct('Selected','no','Byte0','0x00','Byte1','0x00','Byte2','0x00','Byte3','0x00','Byte4','0x00','Byte5','0x00','Byte6','0x00','Byte7','0x00'),'TriggerPort',struct('Selected','no','TriggerType','rising'),'BoardType','DS4302','BoardNo',1,'ControllerNo',1,'SFcnPortType','Scalar'),'TLCFileName','rtican_tx_message')
      settings: AttributesFormatString=Group Id: RTICAN4\n  SourceProductName=dSPACE RTI CAN Blockset
  Bus Selector : BusSelector  OutputSignals=INPUTS.CAN.AIR1_31.AIR1_31Data.PneumaticSupplyPress,INPUTS.CAN.AIR1_31.AIR1_31Data.ParkingAnd_orTrailerAirPress,INPUTS.CAN.AIR1_31.AIR1_31Data.ServiceBrakeCircuit1AirPress,INPUTS.CAN.AIR1_31.AIR1_31Data.ServiceBrakeCircuit2AirPress,INPUTS.CAN.AIR1_31.AIR1_31Data.AuxEquipmentSupplyPress,INPUTS.CAN.AIR1_31.AIR1_31Data.AirSuspensionSupplyPress,INPUTS.CAN.AIR1_31.AIR1_31Data.AirCompressorStatus,INPUTS.CAN.AIR1_31.AIR1_31Data.PowertrainCircuitAirSupplyPress
  Terminator{,1..3} (4 alike) : Terminator
      settings: InitFcn=|
      | try
      |    MBDS_BlockCallback('Update', gcb);
      | end
  wires:
  AIR1/1 -> Terminator/1
  AIR1/3 -> Terminator2/1
  AIR1/4 -> Terminator3/1
  AIR1/2 -> Terminator1/1
  Data/1 -> Bus Selector/1
  Enable/1 -> AIR1/Enable
  Bus Selector/6 -> AIR1/6  "<AirSuspensionSupplyPress>"
  Bus Selector/8 -> AIR1/8  "<PowertrainCircuitAirSupplyPress>"
  Bus Selector/7 -> AIR1/7  "<AirCompressorStatus>"
  Bus Selector/5 -> AIR1/5  "<AuxEquipmentSupplyPress>"
  Bus Selector/3 -> AIR1/3  "<ServiceBrakeCircuit1AirPress>"
  Bus Selector/1 -> AIR1/1  "<PneumaticSupplyPress>"
  Bus Selector/4 -> AIR1/4  "<ServiceBrakeCircuit2AirPress>"
  Bus Selector/2 -> AIR1/2  "<ParkingAnd_orTrailerAirPress>"
